simulink model "MesurementUnit"  (R2021a)
settings: Solver=ode23t  StartTime=0.0  StopTime=20  MaxStep=1e-5  RelTol=1e-3  AbsTol=1e-3
libraries: eeGeneralControl x4, SignalEditorBlockLib x1
settings Model: PacingRate=1000  Creator=ykamatan  LastModifiedBy=ykamatan
settings SolverCC: AutoScaleAbsTol=off  SolverJacobianMethodControl=SparsePerturbation  DaesscMode=Fast
settings DataIOCC: SaveOutput=off  SaveTime=off
settings DebuggingCC: SymbolicDimsDataTypeCodeGenerationDiagnostic=none  SFMachineParentedDataDiag=warning
settings SFSimCC: CustomCodeUndefinedFunction=UseInterfaceOnly
settings SimscapeCC: SimscapeLogDataHistory=10000

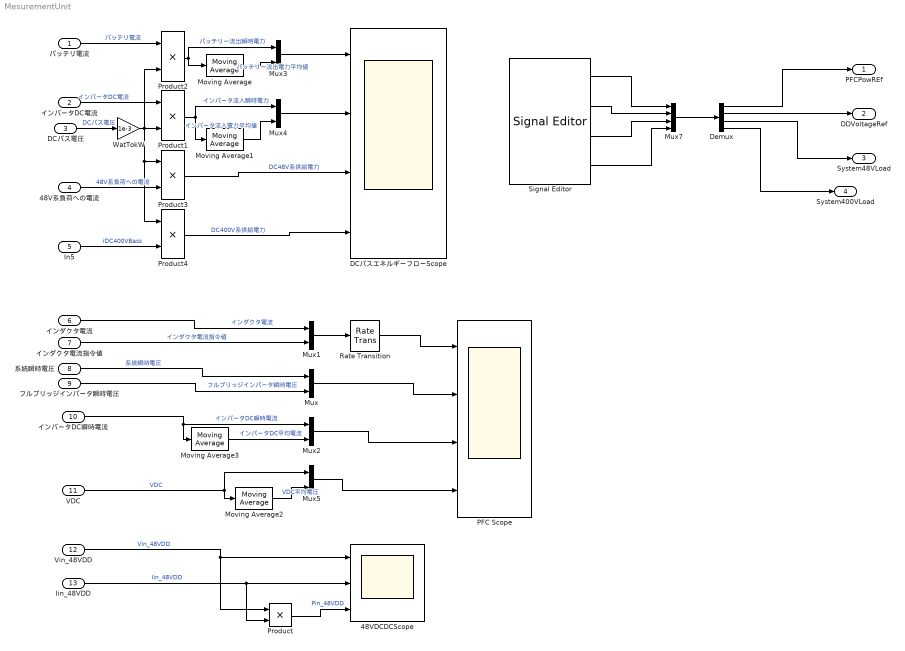
== system MesurementUnit ==
  バッテリ電流 : Inport  OutDataTypeStr=double  PortDimensions=1  SampleTime=0
  インバータDC電流 : Inport  Port=2  OutDataTypeStr=double  PortDimensions=1  SampleTime=0
  DCバス電圧 : Inport  Port=3  OutDataTypeStr=double  PortDimensions=1  SampleTime=0
  48V系負荷への電流 : Inport  Port=4  OutDataTypeStr=double  PortDimensions=1  SampleTime=0
  In5 : Inport  Port=5  OutDataTypeStr=double  PortDimensions=1  SampleTime=0
  インダクタ電流 : Inport  Port=6  OutDataTypeStr=double  PortDimensions=1  SampleTime=0
  インダクタ電流指令値 : Inport  Port=7  OutDataTypeStr=double  PortDimensions=1  SampleTime=[0,1]
  系統瞬時電圧 : Inport  Port=8  OutDataTypeStr=double  PortDimensions=1  SampleTime=0
  フルブリッジインバータ瞬時電圧 : Inport  Port=9  OutDataTypeStr=double  PortDimensions=1  SampleTime=0
  インバータDC瞬時電流 : Inport  Port=10  OutDataTypeStr=double  PortDimensions=1  SampleTime=0
  VDC : Inport  Port=11  OutDataTypeStr=double  PortDimensions=1  SampleTime=0
  Vin_48VDD : Inport  Port=12  OutDataTypeStr=double  PortDimensions=1  SampleTime=0
  Iin_48VDD : Inport  Port=13  OutDataTypeStr=double  PortDimensions=1  SampleTime=0
  48VDCDCScope : Scope  NumInputPorts=3
  DCバスエネルギーフローScope : Scope  NumInputPorts=4
  Demux : Demux
  Moving Average : eeGeneralControl/Moving Average  VariantControl=Variant1  LabelModeActiveChoice=Discrete  f=120  x0=0  Ts=1/120/2
      settings: SourceProductBaseCode=PS
  Moving Average1 : eeGeneralControl/Moving Average  VariantControl=Variant1  LabelModeActiveChoice=Discrete  f=120  x0=0  Ts=1/120/2
      settings: SourceProductBaseCode=PS
  Moving Average2 : eeGeneralControl/Moving Average  VariantControl=Variant1  LabelModeActiveChoice=Discrete  f=120  x0=400  Ts=1/120/2
      settings: SourceProductBaseCode=PS
  Moving Average3 : eeGeneralControl/Moving Average  VariantControl=Variant1  LabelModeActiveChoice=Discrete  f=120  x0=0  Ts=1/120/2
      settings: SourceProductBaseCode=PS
  Mux{,1..5} (6 alike) : Mux  Inputs=2
  Mux7 : Mux
  PFC Scope : Scope  NumInputPorts=4
  Product{,1..4} (5 alike) : Product
  Rate Transition : RateTransition
  Signal Editor : SignalEditorBlockLib/Signal Editor  FileName=InputSignal.mat  ActiveScenario=Scenario  ActiveSignal=PFC_PowerRef  IsBus=off  OutputBusObjectStr=Bus: BusObject  SampleTime=-1  ZeroCross=off  OutputAfterFinalValue=Setting to zero  Unit=inherit  PreserveSignalName=on
  WatTokW : Gain  Gain=1e-3
  PFCPowREf : Outport  OutDataTypeStr=double  PortDimensions=1  SampleTime=0
  DDVoltageRef : Outport  Port=2  OutDataTypeStr=double  PortDimensions=1  SampleTime=0
  System48VLoad : Outport  Port=3
  System400VLoad : Outport  Port=4
  wires:
  Product1/1 -> Moving Average1/1, Mux4/1  "インバータ流入瞬時電力"
  Iin_48VDD/1 -> 48VDCDCScope/2, Product/2  "Iin_48VDD"
  Mux/1 -> PFC Scope/2
  Moving Average/1 -> Mux3/2  "バッテリー流出電力平均値"
  Vin_48VDD/1 -> 48VDCDCScope/1, Product/1  "Vin_48VDD"
  Product/1 -> 48VDCDCScope/3  "Pin_48VDD"
  WatTokW/1 -> Product4/1, Product3/1, Product1/2, Product2/2
  Mux2/1 -> PFC Scope/3
  Product4/1 -> DCバスエネルギーフローScope/4  "DC400V系供給電力"
  インバータDC瞬時電流/1 -> Mux2/1, Moving Average3/1  "インバータDC瞬時電流"
  Mux1/1 -> Rate Transition/1
  Product3/1 -> DCバスエネルギーフローScope/3  "DC48V系供給電力"
  Mux3/1 -> DCバスエネルギーフローScope/1
  Moving Average1/1 -> Mux4/2  "インバータ流入電力平均値"
  Moving Average3/1 -> Mux2/2  "インバータDC平均電流"
  フルブリッジインバータ瞬時電圧/1 -> Mux/2  "フルブリッジインバータ瞬時電圧"
  VDC/1 -> Mux5/1, Moving Average2/1  "VDC"
  Mux5/1 -> PFC Scope/4
  Mux4/1 -> DCバスエネルギーフローScope/2
  インダクタ電流/1 -> Mux1/1  "インダクタ電流"
  Moving Average2/1 -> Mux5/2  "VDC平均電圧"
  Product2/1 -> Moving Average/1, Mux3/1  "バッテリー流出瞬時電力"
  インダクタ電流指令値/1 -> Mux1/2  "インダクタ電流指令値"
  系統瞬時電圧/1 -> Mux/1  "系統瞬時電圧"
  DCバス電圧/1 -> WatTokW/1  "DCバス電圧"
  バッテリ電流/1 -> Product2/1  "バッテリ電流"
  48V系負荷への電流/1 -> Product3/2  "48V系負荷への電流"
  インバータDC電流/1 -> Product1/1  "インバータDC電流"
  In5/1 -> Product4/2  "iDC400VBass"
  Mux7/1 -> Demux/1
  Demux/1 -> PFCPowREf/1
  Demux/2 -> DDVoltageRef/1
  Demux/3 -> System48VLoad/1
  Demux/4 -> System400VLoad/1
  Signal Editor/1 -> Mux7/1
  Signal Editor/3 -> Mux7/3
  Signal Editor/2 -> Mux7/2
  Signal Editor/4 -> Mux7/4
  Rate Transition/1 -> PFC Scope/1
